simulink model "spiBitbang_complete_v2_3_pi"  (R2013b)
settings: Solver=FixedStepDiscrete  StartTime=0.0  StopTime=10  RelTol=1e-3
StopFcn:
  | %run('spiBitBanging_process.m')
model workspace (MAT data in the model file):
  Ts = 0.001
  periSam = 20
undefined symbols (not defined in the file or in its folder): rxdata
libraries: simulink_extras x16, simulink x6, embdlinuxlib x4, dspswit3 x2, dspsnks4 x1
settings Model: VariantConfigurationObject=RxSubsystem  ExtModeTrigDuration=100  Creator=mainster  LastModifiedBy=mainster
settings OptimizationCC: OptimizeModelRefInitCode=on  LifeSpan=1
settings DebuggingCC: SolverPrmCheckMsg=none  UniqueDataStoreMsg=warning  AssertControl=DisableAll
settings HardwareCC: ProdLargestAtomicInteger=Long  ProdLargestAtomicFloat=Double  ProdEndianess=LittleEndian  ProdHWDeviceType=ARM Compatible->ARM Cortex
settings RTWCC: SystemTargetFile=realtime.tlc  GenerateMakefile=off  TemplateMakefile=realtime.tmf  Description=Run on Target Hardware  RTWVerbose=off  ProcessScript=realtime_make_rtw_hook
settings STFCustomTargetCC: TargetLibSuffix=.a  GenerateSampleERTMain=on  ERTCustomFileBanners=on  SupportNonInlinedSFcns=off  SupportVariableSizeSignals=on  MATLABClassNameForMDSCustomization=Simulink.SoftwareTarget.ERTCustomization  GRTInterface=off  SystemTargetFile=realtime.tlc
settings ERTTargetCC: CodeReplacementLibrary=ANSI_C  GenerateSampleERTMain=on  ParMdlRefBuildCompliant=off  CompOptLevelCompliant=off  ConcurrentExecutionCompliant=off  CombineOutputUpdateFcns=off  ERTFirstTimeCompliant=off  SupportContinuousTime=on  SupportVariableSizeSignals=on  ModelStepFunctionPrototypeControlCompliant=off  CPPClassGenCompliant=off  ExtModeMexArgs='192.168.2.111' 0 17725  InlinedParameterPlacement=NonHierarchical  ERTSrcFileBannerTemplate=realtime_code_template.cgt  ERTHdrFileBannerTemplate=realtime_code_template.cgt  ERTDataSrcFileTemplate=realtime_code_template.cgt  ERTDataHdrFileTemplate=realtime_code_template.cgt  ERTCustomFileTemplate=realtime_file_process.tlc
settings SimscapeCC: SelectedTab=Simscape
settings ConfigurationSet: Description=SimMechanics 2G

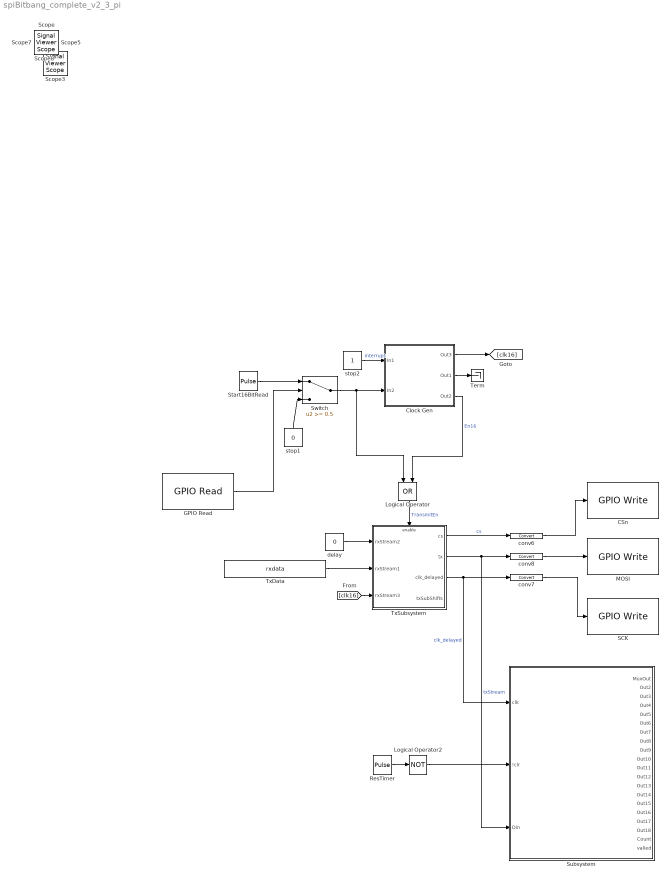
== system spiBitbang_complete_v2_3_pi ==
  CSn : embdlinuxlib/GPIO Write  board=Model B Rev2  gpio=8  direction=Output  blockPlatform=Raspberry Pi
  Clock Gen : Subsystem
  GPIO Read : embdlinuxlib/GPIO Read  board=Model B Rev2  gpio=9  internalResistor=Off  sampleTime=Ts  direction=Input  blockPlatform=Raspberry Pi
  Logical Operator : Logic  Operator=OR  AllPortsSameDT=off  OutDataTypeStr=boolean
  Logical Operator2 : Logic  Operator=NOT  IconShape=distinctive  AllPortsSameDT=off  OutDataTypeStr=boolean
  MOSI : embdlinuxlib/GPIO Write  board=Model B Rev2  gpio=10  direction=Output  blockPlatform=Raspberry Pi
  "ResTimer " : DiscretePulseGenerator  Period=1200  PulseWidth=50  PhaseDelay=70  SampleTime=Ts
  SCK : embdlinuxlib/GPIO Write  board=Model B Rev2  gpio=11  direction=Output  blockPlatform=Raspberry Pi
  Start16BitRead : DiscretePulseGenerator  Period=50000  PulseWidth=20000  PhaseDelay=100  SampleTime=Ts
  Subsystem : Subsystem
  Switch : Switch  Threshold=0.5
  Term : Terminator
  TxData : Constant  Value=rxdata  OutDataTypeStr=uint16  SampleTime=Ts
  TxSubsystem : Subsystem  InitFcn=|
      | set_param('spiBitbang_complete_v2_3_pi/TxSubsystem/cs/','InitialOutput','1')
      | set_param('spiBitbang_complete_v2_3_pi/TxSubsystem/tx/','InitialOutput','0')
      | set_param('spiBitbang_complete_v2_3_pi/TxSubsystem/txSubShifts','InitialOutput','0')
      | set_param('spiBitbang_complete_v2_3_pi/TxSubsystem/clk_delayed','InitialOutput','0')
      settings: PropExecContextOutsideSubsystem=on
  conv6 : DataTypeConversion  LockScale=on
  conv7 : DataTypeConversion  LockScale=on
  conv8 : DataTypeConversion  LockScale=on
  delay : Constant  Value=0  SampleTime=Ts
  stop1 : Constant  Value=0  OutDataTypeStr=Inherit: Inherit via back propagation  SampleTime=Ts
  stop2 : Constant  OutDataTypeStr=Inherit: Inherit via back propagation  SampleTime=Ts
  Scope : SignalViewerScope  IOType=viewer  NumInputPorts=3  RefreshTime=0.035000
      settings: ShowLegends=on  TimeRange=0.0005  YMin=-5~-5~-5  YMax=5~5~5
  Scope3 : SignalViewerScope  IOType=viewer  RefreshTime=0.035000
  Scope5 : SignalViewerScope  IOType=viewer  NumInputPorts=3  LegendLocations=|  RefreshTime=0.035000
      | 0.82061     0.88408     0.20293    0.077088
      | 0.87358     0.60048     0.13389     0.04354
      | 0.82864     0.29053     0.19247     0.04354
      settings: ShowLegends=on  TimeRange=0.0006  YMin=-5~-5~-5  YMax=5~5~5  SaveName=ScopeData2
  Scope7 : SignalViewerScope  IOType=viewer  LegendLocations="0.83596      0.7245     0.13305     0.16299"  RefreshTime=0.035000
      settings: ShowLegends=on  TimeRange=0.0011  YMin=-0.2  YMax=3.5  SaveName=ScopeData4
  Scope8 : SignalViewerScope  IOType=viewer  LegendLocations="0.85063     0.85718     0.13567    0.083065"  RefreshTime=0.035000
      settings: ShowLegends=on  SaveName=ScopeData5
  wires:
  stop2/1 -> Clock Gen/1(In1)  "interrupt"
  Clock Gen/1(Out3) -> [clk16]
  delay/1 -> TxSubsystem/1(rxStream2)
  Clock Gen/2(Out1) -> Term/1
  [clk16] -> TxSubsystem/3(rxStream3)
  Logical Operator/1 -> TxSubsystem/Enable  "TransmitEn"
  Start16BitRead/1 -> Switch/1
  Switch/1 -> Logical Operator/1, Clock Gen/2(In2)
  Clock Gen/3(Out2) -> Logical Operator/2  "En16"
  TxSubsystem/2(tx) -> Subsystem/3(Din), conv8/1  "txStream"
  TxSubsystem/3(clk_delayed) -> Subsystem/1(clk), conv7/1  "clk_delayed"
  "ResTimer "/1 -> Logical Operator2/1
  TxData/1 -> TxSubsystem/2(rxStream1)
  TxSubsystem/1(cs) -> conv6/1  "cs"
  GPIO Read/1 -> Switch/2
  stop1/1 -> Switch/3
  conv6/1 -> CSn/1
  conv7/1 -> SCK/1
  conv8/1 -> MOSI/1
  Logical Operator2/1 -> Subsystem/2(!clr)

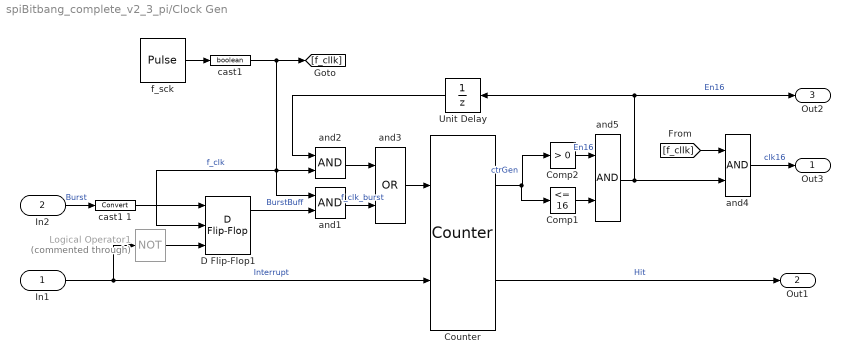
== system spiBitbang_complete_v2_3_pi/Clock Gen ==
  In1 : Inport
  In2 : Inport  Port=2
  Comp1 : simulink/Logic and Bit Operations/Compare To Constant  relop=<=  const=16  OutDataTypeStr=boolean
  Comp2 : simulink/Logic and Bit Operations/Compare To Constant  relop=>  const=0  OutDataTypeStr=boolean
  Counter : dspswit3/Counter  Direction=Up  CountEvent=Rising edge  CounterSize=User defined  MaxCount=16  InitialCount=0  Output=Count and Hit  HitValue=periSam/4  ResetInput=on  SamplesPerFrame=1  Ts=1  CntDtype=double  HitDtype=Logical
  D Flip-Flop1 : simulink_extras/Flip Flops/D Flip-Flop
  Logical Operator1 : Logic  Commented=through  Operator=NOT  IconShape=distinctive  AllPortsSameDT=off  OutDataTypeStr=boolean
  Unit Delay : UnitDelay  SampleTime=-1
  and{1..2,4..5} (4 alike) : Logic  AllPortsSameDT=off  OutDataTypeStr=boolean
      settings: AttributesFormatString=%<Tag>
  and3 : Logic  Operator=OR  AllPortsSameDT=off  OutDataTypeStr=boolean
      settings: AttributesFormatString=%<Tag>
  "cast1 " : DataTypeConversion  OutDataTypeStr=boolean
  cast1 1 : DataTypeConversion
  f_sck : DiscretePulseGenerator  Period=periSam  PulseWidth=periSam/2  SampleTime=Ts
      settings: AttributesFormatString=|
      | Period =%<Period>
      | sTime=%<SampleTime>
      | Delay=%<PhaseDelay>
  Out3 : Outport
  Out1 : Outport  Port=2
  Out2 : Outport  Port=3
  wires:
  "cast1 "/1 -> and1/1, D Flip-Flop1/2, and2/2, [f_cllk]  "f_clk"
  f_sck/1 -> "cast1 "/1
  In1/1 -> Logical Operator1/1, Counter/2  "Interrupt"
  and3/1 -> Counter/1
  and4/1 -> Out3/1  "clk16"
  and1/1 -> and3/2  "f_clk_burst"
  and2/1 -> and3/1
  Unit Delay/1 -> and2/1
  Counter/2 -> Out1/1  "Hit"
  [f_cllk] -> and4/1
  Counter/1 -> Comp1/1, Comp2/1  "ctrGen"
  and5/1 -> Unit Delay/1, Out2/1, and4/2  "En16"
  Comp2/1 -> and5/1  "En16"
  Comp1/1 -> and5/2
  cast1 1/1 -> D Flip-Flop1/1
  Logical Operator1/1 -> D Flip-Flop1/3
  In2/1 -> cast1 1/1  "Burst"
  D Flip-Flop1/1 -> and1/2  "BurstBuff"

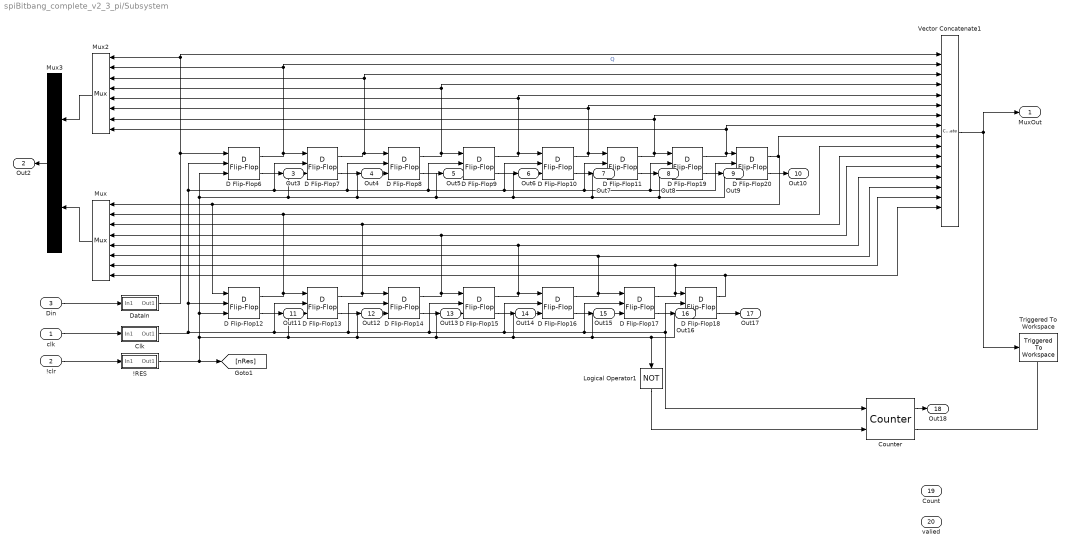
== system spiBitbang_complete_v2_3_pi/Subsystem ==
  clk : Inport
  !clr : Inport  Port=2
  Din : Inport  Port=3
  !RES : Subsystem
  Clk : Subsystem
  Counter : dspswit3/Counter  Direction=Up  CountEvent=Rising edge  CounterSize=User defined  MaxCount=255  InitialCount=0  Output=Count and Hit  HitValue=[15 16 30 31 32]  ResetInput=on  SamplesPerFrame=1  Ts=1  CntDtype=double  HitDtype=Logical
  D Flip-Flop{6..20} (15 alike) : simulink_extras/Flip Flops/D Flip-Flop
  DataIn : Subsystem
  Logical Operator1 : Logic  Operator=NOT  IconShape=distinctive  AllPortsSameDT=off  OutDataTypeStr=boolean
  Mux : Mux  Inputs=8
  Mux2 : Mux  Inputs=8
  Mux3 : Mux  Inputs=2
  Triggered To Workspace : dspsnks4/Triggered To Workspace  TriggerType=Rising edge  VariableName=RxDataRaw  Buffer=1000  Save2DMode=2-D array (concatenate along first dimension)
      settings: FixptAsFi=off
  Vector Concatenate1 : Concatenate  NumInputs=16
  MuxOut : Outport
  Out2 : Outport  Port=2
  Out3 : Outport  Port=3
  Out4 : Outport  Port=4
  Out5 : Outport  Port=5
  Out6 : Outport  Port=6
  Out7 : Outport  Port=7
  Out8 : Outport  Port=8
  Out9 : Outport  Port=9
  Out10 : Outport  Port=10
  Out11 : Outport  Port=11
  Out12 : Outport  Port=12
  Out13 : Outport  Port=13
  Out14 : Outport  Port=14
  Out15 : Outport  Port=15
  Out16 : Outport  Port=16
  Out17 : Outport  Port=17
  Out18 : Outport  Port=18
  Count : Outport  Port=19
  valied : Outport  Port=20
  wires:
  Clk/1(Out1) -> D Flip-Flop14/2, D Flip-Flop15/2, D Flip-Flop18/2, Counter/1, D Flip-Flop17/2, D Flip-Flop16/2, D Flip-Flop13/2, D Flip-Flop12/2, D Flip-Flop7/2, D Flip-Flop8/2, D Flip-Flop9/2, D Flip-Flop10/2, D Flip-Flop11/2, D Flip-Flop19/2, D Flip-Flop20/2, D Flip-Flop6/2
  DataIn/1(Out1) -> Vector Concatenate1/1, Mux2/1, D Flip-Flop6/1
  D Flip-Flop10/2 -> Out7/1
  D Flip-Flop12/2 -> Out11/1
  D Flip-Flop16/2 -> Out15/1
  D Flip-Flop7/2 -> Out4/1
  D Flip-Flop9/2 -> Out6/1
  D Flip-Flop8/2 -> Out5/1
  D Flip-Flop11/2 -> Out8/1
  D Flip-Flop6/2 -> Out3/1
  D Flip-Flop13/2 -> Out12/1
  D Flip-Flop17/2 -> Out16/1
  D Flip-Flop20/2 -> Out10/1
  D Flip-Flop19/2 -> Out9/1
  D Flip-Flop18/2 -> Out17/1
  D Flip-Flop14/2 -> Out13/1
  D Flip-Flop15/2 -> Out14/1
  D Flip-Flop19/1 -> D Flip-Flop20/1, Vector Concatenate1/8, Mux2/8
  Mux2/1 -> Mux3/1
  D Flip-Flop20/1 -> Mux/1, D Flip-Flop12/1, Vector Concatenate1/9
  D Flip-Flop12/1 -> D Flip-Flop13/1, Vector Concatenate1/10, Mux/2
  Mux/1 -> Mux3/2
  D Flip-Flop15/1 -> D Flip-Flop16/1, Mux/5, Vector Concatenate1/13
  D Flip-Flop9/1 -> D Flip-Flop10/1, Vector Concatenate1/5, Mux2/5
  D Flip-Flop6/1 -> D Flip-Flop7/1, Mux2/2, Vector Concatenate1/2  "Q"
  D Flip-Flop18/1 -> Mux/8, Vector Concatenate1/16
  D Flip-Flop14/1 -> D Flip-Flop15/1, Mux/4, Vector Concatenate1/12
  D Flip-Flop10/1 -> D Flip-Flop11/1, Vector Concatenate1/6, Mux2/6
  D Flip-Flop8/1 -> D Flip-Flop9/1, Mux2/4, Vector Concatenate1/4
  D Flip-Flop11/1 -> D Flip-Flop19/1, Mux2/7, Vector Concatenate1/7
  D Flip-Flop17/1 -> D Flip-Flop18/1, Mux/7, Vector Concatenate1/15
  D Flip-Flop16/1 -> D Flip-Flop17/1, Mux/6, Vector Concatenate1/14
  D Flip-Flop13/1 -> D Flip-Flop14/1, Vector Concatenate1/11, Mux/3
  D Flip-Flop7/1 -> D Flip-Flop8/1, Vector Concatenate1/3, Mux2/3
  Vector Concatenate1/1 -> MuxOut/1, Triggered To Workspace/1
  clk/1 -> Clk/1(In1)
  Din/1 -> DataIn/1(In1)
  !clr/1 -> !RES/1(In1)
  !RES/1(Out1) -> [nRes], D Flip-Flop13/3, D Flip-Flop14/3, D Flip-Flop15/3, D Flip-Flop16/3, D Flip-Flop17/3, Logical Operator1/1, D Flip-Flop18/3, D Flip-Flop12/3, D Flip-Flop7/3, D Flip-Flop8/3, D Flip-Flop9/3, D Flip-Flop10/3, D Flip-Flop11/3, D Flip-Flop20/3, D Flip-Flop19/3, D Flip-Flop6/3
  Logical Operator1/1 -> Counter/2
  Counter/2 -> Triggered To Workspace/Trigger
  Counter/1 -> Out18/1
  Mux3/1 -> Out2/1

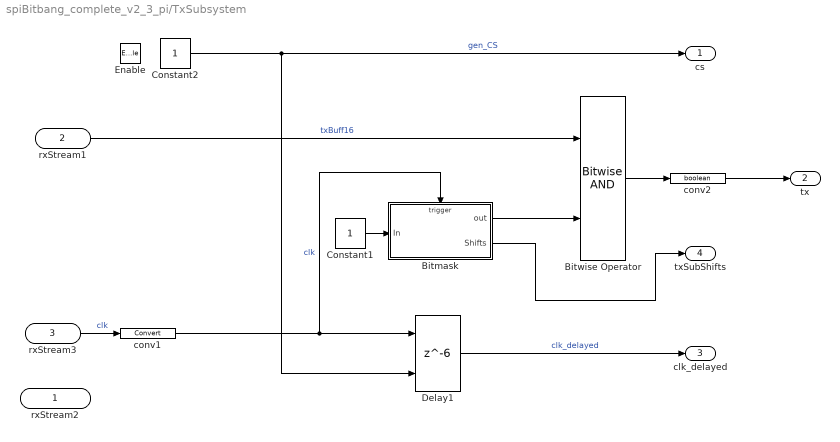
== system spiBitbang_complete_v2_3_pi/TxSubsystem ==
  rxStream2 : Inport
  rxStream1 : Inport  Port=2  OutDataTypeStr=uint16
  rxStream3 : Inport  Port=3
  Enable : EnablePort  StatesWhenEnabling=reset
  Bitmask : Subsystem  TreatAsAtomicUnit=on
  Bitwise Operator : simulink/Logic and Bit Operations/Bitwise Operator  logicop=AND  UseBitMask=off  NumInputPorts=2  BitMask=bin2dec('11011001')  BitMaskRealWorld=Stored Integer
  Constant1 : Constant
  Constant2 : Constant
  Delay1 : Delay  DelayLength=6  InitialCondition=0  ExternalReset=Rising  InputProcessing=Inherited
      settings: InputPortMap=u0,r5
  conv1 : DataTypeConversion
  conv2 : DataTypeConversion  OutDataTypeStr=boolean
  cs : Outport  OutputWhenDisabled=reset  InitialOutput=1
  tx : Outport  Port=2  OutDataTypeStr=boolean  OutputWhenDisabled=reset  InitialOutput=0  LockScale=on
  clk_delayed : Outport  Port=3  OutputWhenDisabled=reset  InitialOutput=0
  txSubShifts : Outport  Port=4  OutputWhenDisabled=reset  InitialOutput=0
  wires:
  Constant2/1 -> cs/1, Delay1/2  "gen_CS"
  rxStream1/1 -> Bitwise Operator/1  "txBuff16"
  rxStream3/1 -> conv1/1  "clk"
  conv1/1 -> Bitmask/Trigger, Delay1/1  "clk"
  Constant1/1 -> Bitmask/1(In)
  Bitmask/1(out) -> Bitwise Operator/2
  Bitwise Operator/1 -> conv2/1
  Bitmask/2(Shifts) -> txSubShifts/1
  Delay1/1 -> clk_delayed/1  "clk_delayed"
  conv2/1 -> tx/1

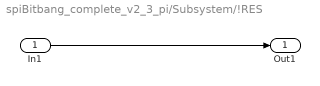
== system spiBitbang_complete_v2_3_pi/Subsystem/!RES ==
  In1 : Inport
  Out1 : Outport
  wires:
  In1/1 -> Out1/1

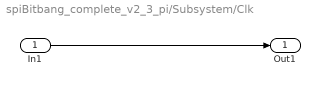
== system spiBitbang_complete_v2_3_pi/Subsystem/Clk ==
  In1 : Inport
  Out1 : Outport
  wires:
  In1/1 -> Out1/1

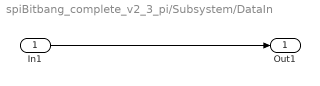
== system spiBitbang_complete_v2_3_pi/Subsystem/DataIn ==
  In1 : Inport
  Out1 : Outport
  wires:
  In1/1 -> Out1/1

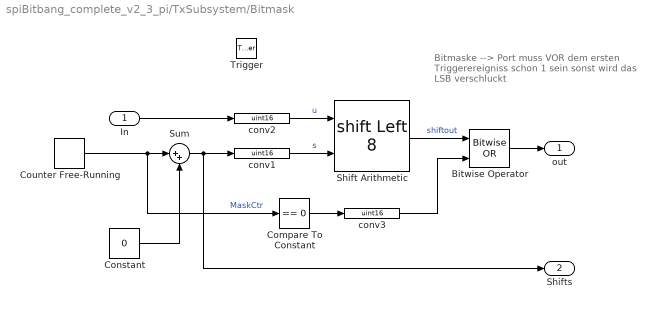
== system spiBitbang_complete_v2_3_pi/TxSubsystem/Bitmask ==
  note: Bitmaske --> Port muss VOR dem ersten
      | Triggerereigniss schon 1 sein sonst wird
      | das LSB verschluckt
  In : Inport
  Trigger : TriggerPort  PortDimensions=1
  Bitwise Operator : simulink/Logic and Bit Operations/Bitwise Operator  logicop=OR  UseBitMask=off  NumInputPorts=2  BitMask=2  BitMaskRealWorld=Stored Integer
  Compare To Constant : simulink/Logic and Bit Operations/Compare To Constant  relop===  const=0  OutDataTypeStr=uint8
  Constant : Constant  Value=0  SampleTime=-1
  Counter Free-Running : simulink/Sources/Counter Free-Running  NumBits=14  tsamp=-1
  Shift Arithmetic : ArithShift  BitShiftNumberSource=Input port  BitShiftNumber=8  BitShiftDirection=Left  DiagnosticForOORShift=Error
      settings: InputPortMap=u0,p1
  Sum : Sum  Inputs=|++
  conv1 : DataTypeConversion  OutDataTypeStr=uint16
  conv2 : DataTypeConversion  OutDataTypeStr=uint16
  conv3 : DataTypeConversion  OutDataTypeStr=uint16
  out : Outport  InitialOutput=[1]
  Shifts : Outport  Port=2
  wires:
  Shift Arithmetic/1 -> Bitwise Operator/1  "shiftout"
  In/1 -> conv2/1
  Sum/1 -> Shifts/1, conv1/1
  Constant/1 -> Sum/2
  conv1/1 -> Shift Arithmetic/2  "s"
  conv2/1 -> Shift Arithmetic/1  "u"
  Counter Free-Running/1 -> Compare To Constant/1, Sum/1  "MaskCtr"
  Bitwise Operator/1 -> out/1
  Compare To Constant/1 -> conv3/1
  conv3/1 -> Bitwise Operator/2
